simulink model "mpc_economicEOWorksheet"  (R2026a)
settings: Solver=ode15s  StopTime=300  MaxStep=5
undefined symbols (not defined in the file or in its folder): u0, x0
settings Model: Creator=The MathWorks, Inc.  LastModifiedBy=GeraldReymariAcobaCa
settings ConfigComp: CovMetricSettings=dsw

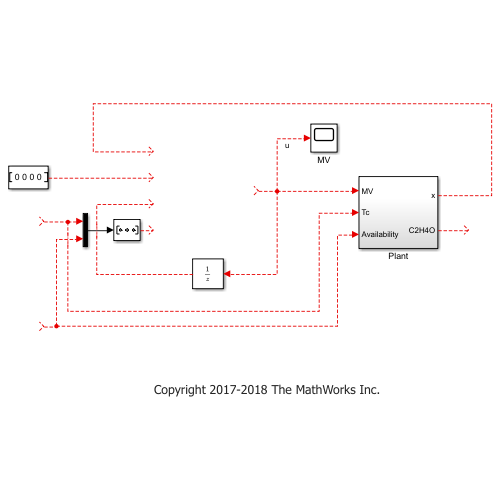
[thumbnail: Simulink's stored preview of the top-level diagram]
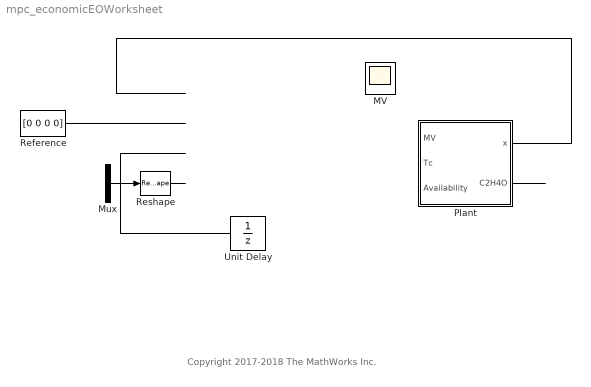
== system mpc_economicEOWorksheet ==
  note: Copyright 2017-2018 The MathWorks Inc.
  MV : Scope
      settings: SampleTime=Ts  ActiveDisplayYMinimum=0.84743  ActiveDisplayYMaximum=2.37309  DataLoggingVariableName=MV  DataLoggingSaveFormat=Array
  Mux : Mux  Inputs=2
  Plant : Subsystem
  Reference : Constant  Value=[0 0 0 0]  VectorParams1D=off
  Reshape : Reshape  OutputDimensionality=Row vector (2-D)
  Unit Delay : UnitDelay  InitialCondition=u0  SampleTime=-1
  wires:
  Plant/1(x) -> ?
  ? -> Plant/2(Tc), Mux/1
  ? -> Unit Delay/1, Plant/1(MV), MV/1  "u"
  Reference/1 -> ?
  Mux/1 -> Reshape/1
  ? -> Mux/2, Plant/3(Availability)
  Plant/2(C2H4O) -> ?
  Reshape/1 -> ?
  Unit Delay/1 -> ?

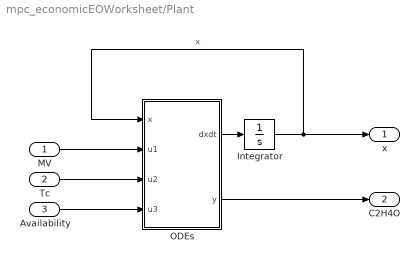
== system mpc_economicEOWorksheet/Plant ==
  MV : Inport
  Tc : Inport  Port=2
  Availability : Inport  Port=3
  Integrator : Integrator  InitialCondition=x0
  ODEs : MATLAB Function  TreatAsAtomicUnit=on
  x : Outport  VectorParamsAs1DForOutWhenUnconnected=off
  C2H4O : Outport  Port=2  VectorParamsAs1DForOutWhenUnconnected=off
  wires:
  Integrator/1 -> ODEs/1(x), x/1  "x"
  ODEs/1(dxdt) -> Integrator/1
  MV/1 -> ODEs/2(u1)
  Tc/1 -> ODEs/3(u2)
  Availability/1 -> ODEs/4(u3)
  ODEs/2(y) -> C2H4O/1

== matlab function mpc_economicEOWorksheet/Plant/ODEs ==
  data: dxdt output; x input; u1 input; u2 input; u3 input; y output
function [dxdt, y] = fcn(x, u1, u2, u3)
% Compute time derivatives and outputs for the ethylene oxide reactor
dxdt = oxidationPlantCT(x, [u1;u2;u3]);
y = u3/u1*x(3)*x(4);
